simulink model "phase_sample_3"  (R2021a)
settings: Solver=VariableStepAuto  StartTime=0.0  StopTime=0.01  RelTol=1e-3
settings Model: Creator=Mrittik  LastModifiedBy=Mrittik

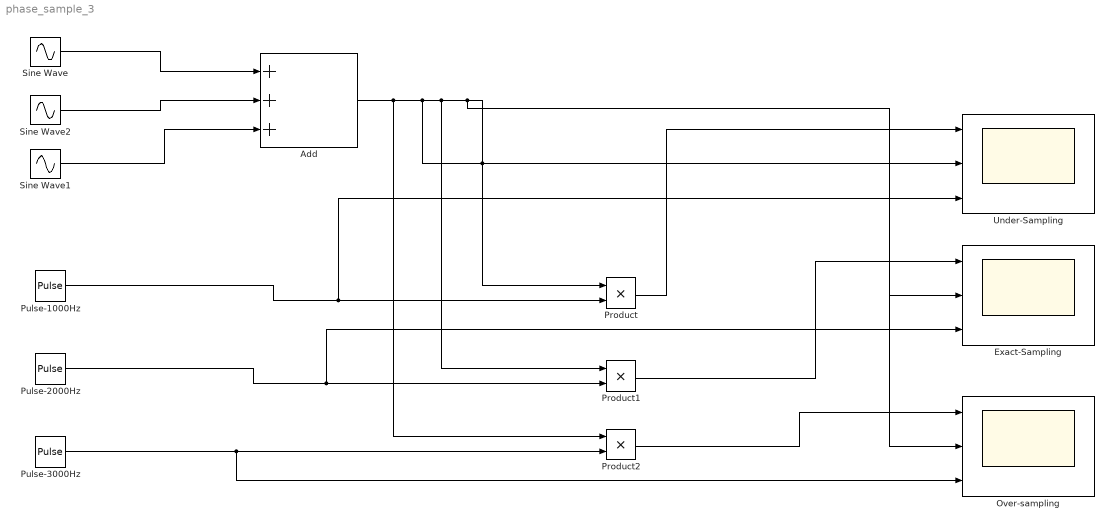
== system phase_sample_3 ==
  Add : Sum  Inputs=+++
  Exact-Sampling : Scope  NumInputPorts=3
  Over-sampling : Scope  NumInputPorts=3
  Product : Product
  Product1 : Product
  Product2 : Product
  Pulse-1000Hz : DiscretePulseGenerator  PulseType=Time based  Period=1/1000  PulseWidth=50
  Pulse-2000Hz : DiscretePulseGenerator  PulseType=Time based  Period=1/2000  PulseWidth=50
  Pulse-3000Hz : DiscretePulseGenerator  PulseType=Time based  Period=1/3000  PulseWidth=50
  Sine Wave : Sin  Frequency=1000  SampleTime=0
  Sine Wave1 : Sin  Frequency=1000  SampleTime=0
  Sine Wave2 : Sin  SampleTime=0
  Under-Sampling : Scope  NumInputPorts=3
  wires:
  Sine Wave/1 -> Add/1
  Sine Wave1/1 -> Add/3
  Add/1 -> Product2/1, Over-sampling/2, Product1/1, Exact-Sampling/2, Under-Sampling/2, Product/1
  Pulse-2000Hz/1 -> Exact-Sampling/3, Product1/2
  Pulse-3000Hz/1 -> Over-sampling/3, Product2/2
  Product/1 -> Under-Sampling/1
  Product1/1 -> Exact-Sampling/1
  Product2/1 -> Over-sampling/1
  Pulse-1000Hz/1 -> Under-Sampling/3, Product/2
  Sine Wave2/1 -> Add/2
